simulink model "Elevation_system"  (R2022b)
settings: Solver=VariableStepAuto  StartTime=0.0  StopTime=30  RelTol=1e-3
model workspace: external: MAT-File /Volumes/GoogleDrive-109291776148936580851/תיקיות אחסון שיתופי/פרויקט גמר/שלב א'/Project_main/Workspace_Project.mat (data not in the file)
libraries: slctrlblks x2
(part 2 of 2)

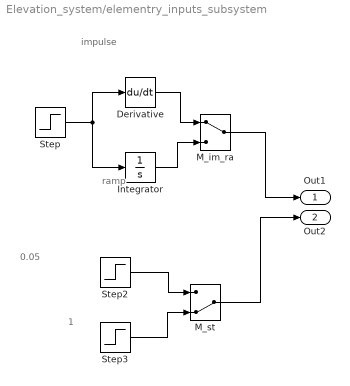
== system Elevation_system/elementry_inputs_subsystem ==
  note: impulse
  note: ramp
  note: 0.05
  note: 1
  Derivative : Derivative
  Integrator : Integrator
  M_im_ra : ManualSwitch
  M_st : ManualSwitch  CurrentSetting=0
  Step : Step  SampleTime=0
  Step2 : Step  After=0.05  SampleTime=0
  Step3 : Step  SampleTime=0
  Out1 : Outport
  Out2 : Outport  Port=2
  wires:
  M_st/1 -> Out2/1
  Step3/1 -> M_st/2
  Derivative/1 -> M_im_ra/1
  M_im_ra/1 -> Out1/1
  Step/1 -> Integrator/1, Derivative/1
  Step2/1 -> M_st/1
  Integrator/1 -> M_im_ra/2
